simulink model "GainScheduledYoula_Estimator_Simulink_J2"  (R2017b)
settings: Solver=VariableStepAuto  StartTime=0.0  StopTime=90000  RelTol=1e-3
InitFcn:
  | load('Sim_Truth_SecondOrder_Corrected5.mat')
  | 
  | load('OCV_table.mat')
values from neighbouring files (symbols this model uses):
  A1 = A(1,1)    [GainScheduledYoula_Code.m]
  A2 = A(2,2)    [GainScheduledYoula_Code.m]
  B1 = B(1,1)    [GainScheduledYoula_Code.m]
  B2 = B(2,1)    [GainScheduledYoula_Code.m]
  C2 = C(1,2)    [GainScheduledYoula_Code.m]
  D = -R0    (= -0.1)    [GainScheduledYoula_Code.m]
  Voc0_1 = 2.915    [GainScheduledYoula_Code.m]
  Voc0_2 = 3.4099    [GainScheduledYoula_Code.m]
undefined symbols (not defined in the file or in its folder): den1, den2, num1, num2
libraries: dspsrcs4 x4
settings Model: Creator=Indiana  LastModifiedBy=Indiana
settings SFSimCC: SimUseLocalCustomCode=on
settings RTWCC: RTWUseLocalCustomCode=on

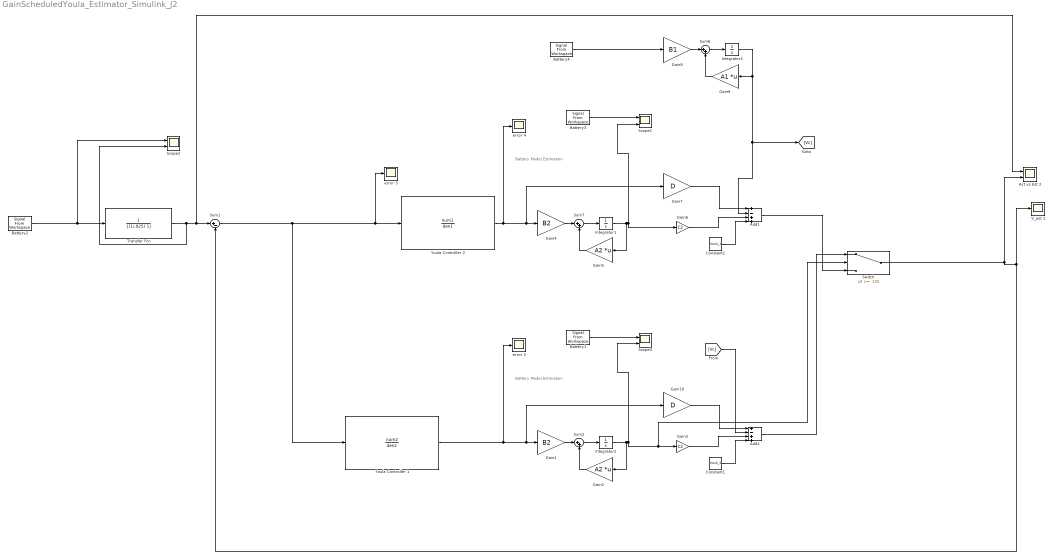
== system GainScheduledYoula_Estimator_Simulink_J2 ==
  note: Battery Model Estimation
  note: Battery Model Estimation
  Act vs Est 2 : Scope  NumInputPorts=2
  Add1 : Sum  Inputs=+-++
  Add2 : Sum  Inputs=+-++
  Battery1 : dspsrcs4/Signal From Workspace  X=SOC_act  Ts=1  nsamps=1  OutputAfterFinalValue=Setting to zero  ignoreOrWarnInputAndFrameLengths=off  OutputFrames=off
  Battery2 : dspsrcs4/Signal From Workspace  X=V  Ts=1  nsamps=1  OutputAfterFinalValue=Setting to zero  ignoreOrWarnInputAndFrameLengths=off  OutputFrames=off
  Battery3 : dspsrcs4/Signal From Workspace  X=SOC_act  Ts=1  nsamps=1  OutputAfterFinalValue=Setting to zero  ignoreOrWarnInputAndFrameLengths=off  OutputFrames=off
  Battery4 : dspsrcs4/Signal From Workspace  X=I  Ts=1  nsamps=1  OutputAfterFinalValue=Setting to zero  ignoreOrWarnInputAndFrameLengths=off  OutputFrames=off
  Constant1 : Constant  Value=Voc0_2
  Constant2 : Constant  Value=Voc0_1
  Gain1 : Gain  Gain=B2
  Gain10 : Gain  Gain=D
  Gain2 : Gain  Gain=A2  Multiplication=Matrix(K*u)
  Gain3 : Gain  Gain=C2
  Gain4 : Gain  Gain=B2
  Gain5 : Gain  Gain=A2  Multiplication=Matrix(K*u)
  Gain6 : Gain  Gain=C2
  Gain7 : Gain  Gain=D
  Gain8 : Gain  Gain=B1
  Gain9 : Gain  Gain=A1  Multiplication=Matrix(K*u)
  Integrator1 : Integrator  InitialCondition=[.98]
  Integrator2 : Integrator  InitialCondition=[.98]
  Integrator3 : Integrator  InitialCondition=[0]
  Scope1 : Scope  NumInputPorts=2
  Scope2 : Scope  NumInputPorts=2
  Scope3 : Scope  NumInputPorts=2
  Sum1 : Sum  Inputs=|+-
  Sum2 : Sum  Inputs=|++
  Sum6 : Sum  Inputs=|++
  Sum7 : Sum  Inputs=|++
  Switch : Switch  Threshold=.125
  Transfer Fcn : TransferFcn  Denominator=[(1/.025) 1]
  V_est 1 : Scope
  Youla Controller 1 : TransferFcn  Numerator=num2  Denominator=den2
  Youla Controller 2 : TransferFcn  Numerator=num1  Denominator=den1
  error 2 : Scope
  error 3 : Scope
  error 4 : Scope
  wires:
  Gain4/1 -> Sum7/1
  Gain5/1 -> Sum7/2
  Sum7/1 -> Integrator1/1
  Youla Controller 2/1 -> Gain7/1, Gain4/1, error 4/1
  Battery3/1 -> Scope1/1
  Gain7/1 -> Add1/1
  Battery2/1 -> Transfer Fcn/1, Scope2/1
  Transfer Fcn/1 -> Scope2/2, Act vs Est 2/1, Sum1/1
  Gain9/1 -> Sum6/2
  Sum6/1 -> Integrator3/1
  Gain8/1 -> Sum6/1
  Battery4/1 -> Gain8/1
  Gain6/1 -> Add1/3
  Constant2/1 -> Add1/4
  Integrator3/1 -> [Vc], Add1/2, Gain9/1
  Gain3/1 -> Add2/3
  Constant1/1 -> Add2/4
  Add2/1 -> Switch/1
  Gain10/1 -> Add2/1
  Battery1/1 -> Scope3/1
  Gain2/1 -> Sum2/2
  Gain1/1 -> Sum2/1
  Sum1/1 -> Youla Controller 1/1, Youla Controller 2/1, error 3/1
  Sum2/1 -> Integrator2/1
  Youla Controller 1/1 -> Gain10/1, Gain1/1, error 2/1
  Switch/1 -> Sum1/2, V_est 1/1, Act vs Est 2/2
  [Vc] -> Add2/2
  Integrator1/1 -> Gain6/1, Scope1/2, Gain5/1
  Integrator2/1 -> Switch/2, Gain3/1, Scope3/2, Gain2/1
  Add1/1 -> Switch/3
